simulink model "nofeedback"  (R2015a)
settings: Solver=ode45  StartTime=0.0  StopTime=10.0  RelTol=1e-3
libraries: cstblocks x3
settings Model: Creator=roevhat  LastModifiedBy=roevhat

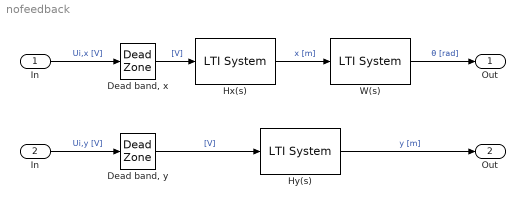
== system nofeedback ==
  In : Inport
  "In " : Inport  Port=2
  "Dead band, x" : DeadZone  LowerValue=4.2  UpperValue=4.2  SaturateOnIntegerOverflow=on
  "Dead band, y" : DeadZone  LowerValue=4.2  UpperValue=4.2  SaturateOnIntegerOverflow=on
  Hx(s) : cstblocks/LTI System  sys=Hx  IC=[]
  Hy(s) : cstblocks/LTI System  sys=Hy  IC=[]
  W(s) : cstblocks/LTI System  sys=W  IC=[]
  Out : Outport
  "Out " : Outport  Port=2
  wires:
  Hx(s)/1 -> W(s)/1  "x [m]"
  "Dead band, x"/1 -> Hx(s)/1  "[V]"
  W(s)/1 -> Out/1  "θ [rad]"
  In/1 -> "Dead band, x"/1  "Ui,x [V]"
  Hy(s)/1 -> "Out "/1  "y [m]"
  "Dead band, y"/1 -> Hy(s)/1  "[V]"
  "In "/1 -> "Dead band, y"/1  "Ui,y [V]"
